simulink model "DFADAS2_SenFus_v1_201204RC_training_210115"  (R2018b)
settings: Solver=FixedStepDiscrete  StartTime=0.0  StopTime=inf  FixedStep=0.002  RelTol=1e-3  EnableMultiTasking=on
PreLoadFcn:
  | RTWConfigurationCB('preloadfcn', bdroot);
libraries: canmsglib x108, simulink x48, canfdmsglib x12
(part 2 of 28)

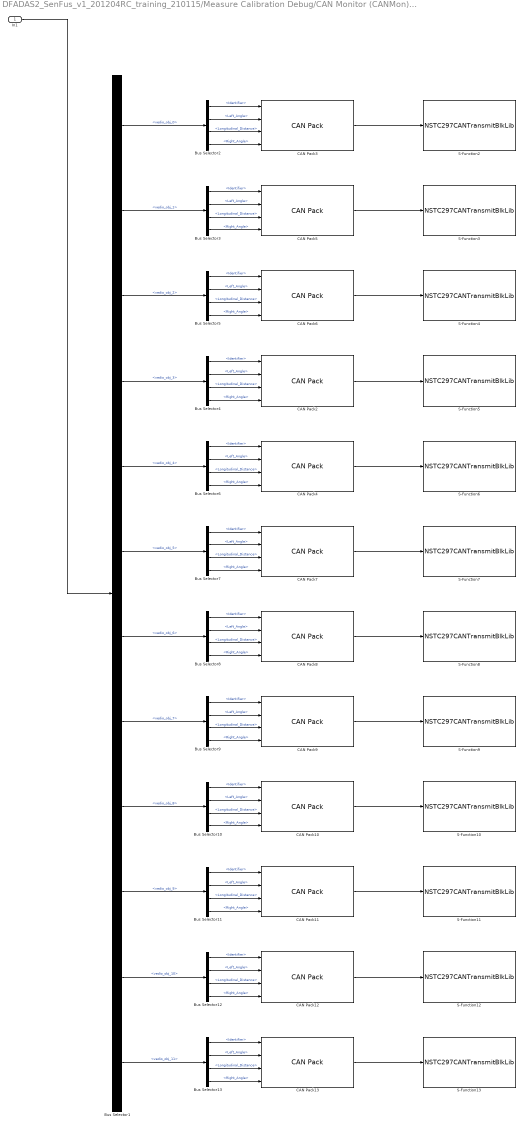
== system DFADAS2_SenFus_v1_201204RC_training_210115/Measure Calibration Debug/CAN Monitor (CANMon)/CamObjinfo ==
  In1 : Inport
  Bus Selector1 : BusSelector  OutputSignals=RawIn_bsInInfo50.EnvSens.RawObjInfo.CmrFrt.vedio_obj_0,RawIn_bsInInfo50.EnvSens.RawObjInfo.CmrFrt.vedio_obj_1,RawIn_bsInInfo50.EnvSens.RawObjInfo.CmrFrt.vedio_obj_2,RawIn_bsInInfo50.EnvSens.RawObjInfo.CmrFrt.vedio_obj_3,RawIn_bsInInfo50.EnvSens.RawObjInfo.CmrFrt.vedio_obj_4,RawIn_bsInInfo50.EnvSens.RawObjInfo.CmrFrt.vedio_obj_5,RawIn_bsInInfo50.EnvSens.RawObjInfo.CmrFrt.vedio_obj_6,RawIn_bsInInfo50.EnvSens.RawObjInfo.CmrFrt.vedio_obj_7,RawIn_bsInInfo50.EnvSens.RawObjInfo.CmrFrt.vedio_obj_8,RawIn_bsInInfo50.EnvSens.RawObjInfo.CmrFrt.vedio_obj_9,RawIn_bsInInfo50.EnvSens.RawObjInfo.CmrFrt.vedio_obj_10,RawIn_bsInInfo50.EnvSens.RawObjInfo.CmrFrt.vedio_obj_11
  Bus Selector{2..13} (12 alike) : BusSelector  OutputSignals=Identifier,Left_Angle,Longitudinal_Distance,Right_Angle
  CAN Pack10 : canmsglib/CAN Pack  CANdbFile=D:\work\ADAS ECU-Sensor CAN_V2_20190314(1).dbc  MsgList=(none)  MsgName=Video_Object_0_A  MsgIDType=Standard (11-bit identifier)  MsgIdentifier=1991  MsgLength=8  SignalInfo=Identifier_700$0$16$1$2$1$0$1$0$0$127$#Left_Angle_700$16$16$1$1$1$0$2.000000e-04$0$-8.192000e-01$8.190000e-01$#Longitudinal_Distance_700$32$16$1$2$1$0$5.000000e-02$0$0$2.047500e+02$#Right_Angle_700$48$16$1$1$1$0$2.000000e-04$0$-8.192000e-01$8.190000e-01$#  NSignals=4  StartBits=str2num('[int32(0);int32(16);int32(32);int32(48)]')  SignalSizes=str2num('[int32(16);int32(16);int32(16);int32(16)]')  ByteOrders=str2num('[int32(1);int32(1);int32(1);int32(1)]')  DataTypes=str2num('[int32(2);int32(1);int32(2);int32(1)]')  MultiplexTypes=str2num('[int32(1);int32(1);int32(1);int32(1)]')  MultiplexValues=str2num('[double(0);double(0);double(0);double(0)]')  Factors=str2num('[double(1);double(2.000000e-04);double(5.000000e-02);double(2.000000e-04)]')  Offsets=str2num('[double(0);double(0);double(0);double(0)]')  Minimums=str2num('[double(0);double(-8.192000e-01);double(0);double(-8.192000e-01)]')  Maximums=str2num('[double(127);double(8.190000e-01);double(2.047500e+02);double(8.190000e-01)]')  Remote=off  ApplyMinMax=off  BusOutput=on
      settings: SourceProductName=Simulink Real-Time  SourceProductBaseCode=XP  DataFormat=manually specified signals
  CAN Pack11 : canmsglib/CAN Pack  CANdbFile=D:\work\ADAS ECU-Sensor CAN_V2_20190314(1).dbc  MsgList=(none)  MsgName=Video_Object_0_A  MsgIDType=Standard (11-bit identifier)  MsgIdentifier=1990  MsgLength=8  SignalInfo=Identifier_700$0$16$1$2$1$0$1$0$0$127$#Left_Angle_700$16$16$1$1$1$0$2.000000e-04$0$-8.192000e-01$8.190000e-01$#Longitudinal_Distance_700$32$16$1$2$1$0$5.000000e-02$0$0$2.047500e+02$#Right_Angle_700$48$16$1$1$1$0$2.000000e-04$0$-8.192000e-01$8.190000e-01$#  NSignals=4  StartBits=str2num('[int32(0);int32(16);int32(32);int32(48)]')  SignalSizes=str2num('[int32(16);int32(16);int32(16);int32(16)]')  ByteOrders=str2num('[int32(1);int32(1);int32(1);int32(1)]')  DataTypes=str2num('[int32(2);int32(1);int32(2);int32(1)]')  MultiplexTypes=str2num('[int32(1);int32(1);int32(1);int32(1)]')  MultiplexValues=str2num('[double(0);double(0);double(0);double(0)]')  Factors=str2num('[double(1);double(2.000000e-04);double(5.000000e-02);double(2.000000e-04)]')  Offsets=str2num('[double(0);double(0);double(0);double(0)]')  Minimums=str2num('[double(0);double(-8.192000e-01);double(0);double(-8.192000e-01)]')  Maximums=str2num('[double(127);double(8.190000e-01);double(2.047500e+02);double(8.190000e-01)]')  Remote=off  ApplyMinMax=off  BusOutput=on
      settings: SourceProductName=Simulink Real-Time  SourceProductBaseCode=XP  DataFormat=manually specified signals
  CAN Pack12 : canmsglib/CAN Pack  CANdbFile=D:\work\ADAS ECU-Sensor CAN_V2_20190314(1).dbc  MsgList=(none)  MsgName=Video_Object_0_A  MsgIDType=Standard (11-bit identifier)  MsgIdentifier=1989  MsgLength=8  SignalInfo=Identifier_700$0$16$1$2$1$0$1$0$0$127$#Left_Angle_700$16$16$1$1$1$0$2.000000e-04$0$-8.192000e-01$8.190000e-01$#Longitudinal_Distance_700$32$16$1$2$1$0$5.000000e-02$0$0$2.047500e+02$#Right_Angle_700$48$16$1$1$1$0$2.000000e-04$0$-8.192000e-01$8.190000e-01$#  NSignals=4  StartBits=str2num('[int32(0);int32(16);int32(32);int32(48)]')  SignalSizes=str2num('[int32(16);int32(16);int32(16);int32(16)]')  ByteOrders=str2num('[int32(1);int32(1);int32(1);int32(1)]')  DataTypes=str2num('[int32(2);int32(1);int32(2);int32(1)]')  MultiplexTypes=str2num('[int32(1);int32(1);int32(1);int32(1)]')  MultiplexValues=str2num('[double(0);double(0);double(0);double(0)]')  Factors=str2num('[double(1);double(2.000000e-04);double(5.000000e-02);double(2.000000e-04)]')  Offsets=str2num('[double(0);double(0);double(0);double(0)]')  Minimums=str2num('[double(0);double(-8.192000e-01);double(0);double(-8.192000e-01)]')  Maximums=str2num('[double(127);double(8.190000e-01);double(2.047500e+02);double(8.190000e-01)]')  Remote=off  ApplyMinMax=off  BusOutput=on
      settings: SourceProductName=Simulink Real-Time  SourceProductBaseCode=XP  DataFormat=manually specified signals
  CAN Pack13 : canmsglib/CAN Pack  CANdbFile=D:\work\ADAS ECU-Sensor CAN_V2_20190314(1).dbc  MsgList=(none)  MsgName=Video_Object_0_A  MsgIDType=Standard (11-bit identifier)  MsgIdentifier=1988  MsgLength=8  SignalInfo=Identifier_700$0$16$1$2$1$0$1$0$0$127$#Left_Angle_700$16$16$1$1$1$0$2.000000e-04$0$-8.192000e-01$8.190000e-01$#Longitudinal_Distance_700$32$16$1$2$1$0$5.000000e-02$0$0$2.047500e+02$#Right_Angle_700$48$16$1$1$1$0$2.000000e-04$0$-8.192000e-01$8.190000e-01$#  NSignals=4  StartBits=str2num('[int32(0);int32(16);int32(32);int32(48)]')  SignalSizes=str2num('[int32(16);int32(16);int32(16);int32(16)]')  ByteOrders=str2num('[int32(1);int32(1);int32(1);int32(1)]')  DataTypes=str2num('[int32(2);int32(1);int32(2);int32(1)]')  MultiplexTypes=str2num('[int32(1);int32(1);int32(1);int32(1)]')  MultiplexValues=str2num('[double(0);double(0);double(0);double(0)]')  Factors=str2num('[double(1);double(2.000000e-04);double(5.000000e-02);double(2.000000e-04)]')  Offsets=str2num('[double(0);double(0);double(0);double(0)]')  Minimums=str2num('[double(0);double(-8.192000e-01);double(0);double(-8.192000e-01)]')  Maximums=str2num('[double(127);double(8.190000e-01);double(2.047500e+02);double(8.190000e-01)]')  Remote=off  ApplyMinMax=off  BusOutput=on
      settings: SourceProductName=Simulink Real-Time  SourceProductBaseCode=XP  DataFormat=manually specified signals
  CAN Pack2 : canmsglib/CAN Pack  CANdbFile=D:\work\ADAS ECU-Sensor CAN_V2_20190314(1).dbc  MsgList=(none)  MsgName=Video_Object_0_A  MsgIDType=Standard (11-bit identifier)  MsgIdentifier=1996  MsgLength=8  SignalInfo=Identifier_700$0$16$1$2$1$0$1$0$0$127$#Left_Angle_700$16$16$1$1$1$0$2.000000e-04$0$-8.192000e-01$8.190000e-01$#Longitudinal_Distance_700$32$16$1$2$1$0$5.000000e-02$0$0$2.047500e+02$#Right_Angle_700$48$16$1$1$1$0$2.000000e-04$0$-8.192000e-01$8.190000e-01$#  NSignals=4  StartBits=str2num('[int32(0);int32(16);int32(32);int32(48)]')  SignalSizes=str2num('[int32(16);int32(16);int32(16);int32(16)]')  ByteOrders=str2num('[int32(1);int32(1);int32(1);int32(1)]')  DataTypes=str2num('[int32(2);int32(1);int32(2);int32(1)]')  MultiplexTypes=str2num('[int32(1);int32(1);int32(1);int32(1)]')  MultiplexValues=str2num('[double(0);double(0);double(0);double(0)]')  Factors=str2num('[double(1);double(2.000000e-04);double(5.000000e-02);double(2.000000e-04)]')  Offsets=str2num('[double(0);double(0);double(0);double(0)]')  Minimums=str2num('[double(0);double(-8.192000e-01);double(0);double(-8.192000e-01)]')  Maximums=str2num('[double(127);double(8.190000e-01);double(2.047500e+02);double(8.190000e-01)]')  Remote=off  ApplyMinMax=off  BusOutput=on
      settings: SourceProductName=Simulink Real-Time  SourceProductBaseCode=XP  DataFormat=manually specified signals
  CAN Pack3 : canmsglib/CAN Pack  CANdbFile=D:\work\ADAS ECU-Sensor CAN_V2_20190314(1).dbc  MsgList=(none)  MsgName=Video_Object_0_A  MsgIDType=Standard (11-bit identifier)  MsgIdentifier=1999  MsgLength=8  SignalInfo=Identifier_700$0$16$1$2$1$0$1$0$0$127$#Left_Angle_700$16$16$1$1$1$0$2.000000e-04$0$-8.192000e-01$8.190000e-01$#Longitudinal_Distance_700$32$16$1$2$1$0$5.000000e-02$0$0$2.047500e+02$#Right_Angle_700$48$16$1$1$1$0$2.000000e-04$0$-8.192000e-01$8.190000e-01$#  NSignals=4  StartBits=str2num('[int32(0);int32(16);int32(32);int32(48)]')  SignalSizes=str2num('[int32(16);int32(16);int32(16);int32(16)]')  ByteOrders=str2num('[int32(1);int32(1);int32(1);int32(1)]')  DataTypes=str2num('[int32(2);int32(1);int32(2);int32(1)]')  MultiplexTypes=str2num('[int32(1);int32(1);int32(1);int32(1)]')  MultiplexValues=str2num('[double(0);double(0);double(0);double(0)]')  Factors=str2num('[double(1);double(2.000000e-04);double(5.000000e-02);double(2.000000e-04)]')  Offsets=str2num('[double(0);double(0);double(0);double(0)]')  Minimums=str2num('[double(0);double(-8.192000e-01);double(0);double(-8.192000e-01)]')  Maximums=str2num('[double(127);double(8.190000e-01);double(2.047500e+02);double(8.190000e-01)]')  Remote=off  ApplyMinMax=off  BusOutput=on
      settings: SourceProductName=Simulink Real-Time  SourceProductBaseCode=XP  DataFormat=manually specified signals
  CAN Pack4 : canmsglib/CAN Pack  CANdbFile=D:\work\ADAS ECU-Sensor CAN_V2_20190314(1).dbc  MsgList=(none)  MsgName=Video_Object_0_A  MsgIDType=Standard (11-bit identifier)  MsgIdentifier=1995  MsgLength=8  SignalInfo=Identifier_700$0$16$1$2$1$0$1$0$0$127$#Left_Angle_700$16$16$1$1$1$0$2.000000e-04$0$-8.192000e-01$8.190000e-01$#Longitudinal_Distance_700$32$16$1$2$1$0$5.000000e-02$0$0$2.047500e+02$#Right_Angle_700$48$16$1$1$1$0$2.000000e-04$0$-8.192000e-01$8.190000e-01$#  NSignals=4  StartBits=str2num('[int32(0);int32(16);int32(32);int32(48)]')  SignalSizes=str2num('[int32(16);int32(16);int32(16);int32(16)]')  ByteOrders=str2num('[int32(1);int32(1);int32(1);int32(1)]')  DataTypes=str2num('[int32(2);int32(1);int32(2);int32(1)]')  MultiplexTypes=str2num('[int32(1);int32(1);int32(1);int32(1)]')  MultiplexValues=str2num('[double(0);double(0);double(0);double(0)]')  Factors=str2num('[double(1);double(2.000000e-04);double(5.000000e-02);double(2.000000e-04)]')  Offsets=str2num('[double(0);double(0);double(0);double(0)]')  Minimums=str2num('[double(0);double(-8.192000e-01);double(0);double(-8.192000e-01)]')  Maximums=str2num('[double(127);double(8.190000e-01);double(2.047500e+02);double(8.190000e-01)]')  Remote=off  ApplyMinMax=off  BusOutput=on
      settings: SourceProductName=Simulink Real-Time  SourceProductBaseCode=XP  DataFormat=manually specified signals
  CAN Pack5 : canmsglib/CAN Pack  CANdbFile=D:\work\ADAS ECU-Sensor CAN_V2_20190314(1).dbc  MsgList=(none)  MsgName=Video_Object_0_A  MsgIDType=Standard (11-bit identifier)  MsgIdentifier=1998  MsgLength=8  SignalInfo=Identifier_700$0$16$1$2$1$0$1$0$0$127$#Left_Angle_700$16$16$1$1$1$0$2.000000e-04$0$-8.192000e-01$8.190000e-01$#Longitudinal_Distance_700$32$16$1$2$1$0$5.000000e-02$0$0$2.047500e+02$#Right_Angle_700$48$16$1$1$1$0$2.000000e-04$0$-8.192000e-01$8.190000e-01$#  NSignals=4  StartBits=str2num('[int32(0);int32(16);int32(32);int32(48)]')  SignalSizes=str2num('[int32(16);int32(16);int32(16);int32(16)]')  ByteOrders=str2num('[int32(1);int32(1);int32(1);int32(1)]')  DataTypes=str2num('[int32(2);int32(1);int32(2);int32(1)]')  MultiplexTypes=str2num('[int32(1);int32(1);int32(1);int32(1)]')  MultiplexValues=str2num('[double(0);double(0);double(0);double(0)]')  Factors=str2num('[double(1);double(2.000000e-04);double(5.000000e-02);double(2.000000e-04)]')  Offsets=str2num('[double(0);double(0);double(0);double(0)]')  Minimums=str2num('[double(0);double(-8.192000e-01);double(0);double(-8.192000e-01)]')  Maximums=str2num('[double(127);double(8.190000e-01);double(2.047500e+02);double(8.190000e-01)]')  Remote=off  ApplyMinMax=off  BusOutput=on
      settings: SourceProductName=Simulink Real-Time  SourceProductBaseCode=XP  DataFormat=manually specified signals
  CAN Pack6 : canmsglib/CAN Pack  CANdbFile=D:\work\ADAS ECU-Sensor CAN_V2_20190314(1).dbc  MsgList=(none)  MsgName=Video_Object_0_A  MsgIDType=Standard (11-bit identifier)  MsgIdentifier=1997  MsgLength=8  SignalInfo=Identifier_700$0$16$1$2$1$0$1$0$0$127$#Left_Angle_700$16$16$1$1$1$0$2.000000e-04$0$-8.192000e-01$8.190000e-01$#Longitudinal_Distance_700$32$16$1$2$1$0$5.000000e-02$0$0$2.047500e+02$#Right_Angle_700$48$16$1$1$1$0$2.000000e-04$0$-8.192000e-01$8.190000e-01$#  NSignals=4  StartBits=str2num('[int32(0);int32(16);int32(32);int32(48)]')  SignalSizes=str2num('[int32(16);int32(16);int32(16);int32(16)]')  ByteOrders=str2num('[int32(1);int32(1);int32(1);int32(1)]')  DataTypes=str2num('[int32(2);int32(1);int32(2);int32(1)]')  MultiplexTypes=str2num('[int32(1);int32(1);int32(1);int32(1)]')  MultiplexValues=str2num('[double(0);double(0);double(0);double(0)]')  Factors=str2num('[double(1);double(2.000000e-04);double(5.000000e-02);double(2.000000e-04)]')  Offsets=str2num('[double(0);double(0);double(0);double(0)]')  Minimums=str2num('[double(0);double(-8.192000e-01);double(0);double(-8.192000e-01)]')  Maximums=str2num('[double(127);double(8.190000e-01);double(2.047500e+02);double(8.190000e-01)]')  Remote=off  ApplyMinMax=off  BusOutput=on
      settings: SourceProductName=Simulink Real-Time  SourceProductBaseCode=XP  DataFormat=manually specified signals
  CAN Pack7 : canmsglib/CAN Pack  CANdbFile=D:\work\ADAS ECU-Sensor CAN_V2_20190314(1).dbc  MsgList=(none)  MsgName=Video_Object_0_A  MsgIDType=Standard (11-bit identifier)  MsgIdentifier=1994  MsgLength=8  SignalInfo=Identifier_700$0$16$1$2$1$0$1$0$0$127$#Left_Angle_700$16$16$1$1$1$0$2.000000e-04$0$-8.192000e-01$8.190000e-01$#Longitudinal_Distance_700$32$16$1$2$1$0$5.000000e-02$0$0$2.047500e+02$#Right_Angle_700$48$16$1$1$1$0$2.000000e-04$0$-8.192000e-01$8.190000e-01$#  NSignals=4  StartBits=str2num('[int32(0);int32(16);int32(32);int32(48)]')  SignalSizes=str2num('[int32(16);int32(16);int32(16);int32(16)]')  ByteOrders=str2num('[int32(1);int32(1);int32(1);int32(1)]')  DataTypes=str2num('[int32(2);int32(1);int32(2);int32(1)]')  MultiplexTypes=str2num('[int32(1);int32(1);int32(1);int32(1)]')  MultiplexValues=str2num('[double(0);double(0);double(0);double(0)]')  Factors=str2num('[double(1);double(2.000000e-04);double(5.000000e-02);double(2.000000e-04)]')  Offsets=str2num('[double(0);double(0);double(0);double(0)]')  Minimums=str2num('[double(0);double(-8.192000e-01);double(0);double(-8.192000e-01)]')  Maximums=str2num('[double(127);double(8.190000e-01);double(2.047500e+02);double(8.190000e-01)]')  Remote=off  ApplyMinMax=off  BusOutput=on
      settings: SourceProductName=Simulink Real-Time  SourceProductBaseCode=XP  DataFormat=manually specified signals
  CAN Pack8 : canmsglib/CAN Pack  CANdbFile=D:\work\ADAS ECU-Sensor CAN_V2_20190314(1).dbc  MsgList=(none)  MsgName=Video_Object_0_A  MsgIDType=Standard (11-bit identifier)  MsgIdentifier=1993  MsgLength=8  SignalInfo=Identifier_700$0$16$1$2$1$0$1$0$0$127$#Left_Angle_700$16$16$1$1$1$0$2.000000e-04$0$-8.192000e-01$8.190000e-01$#Longitudinal_Distance_700$32$16$1$2$1$0$5.000000e-02$0$0$2.047500e+02$#Right_Angle_700$48$16$1$1$1$0$2.000000e-04$0$-8.192000e-01$8.190000e-01$#  NSignals=4  StartBits=str2num('[int32(0);int32(16);int32(32);int32(48)]')  SignalSizes=str2num('[int32(16);int32(16);int32(16);int32(16)]')  ByteOrders=str2num('[int32(1);int32(1);int32(1);int32(1)]')  DataTypes=str2num('[int32(2);int32(1);int32(2);int32(1)]')  MultiplexTypes=str2num('[int32(1);int32(1);int32(1);int32(1)]')  MultiplexValues=str2num('[double(0);double(0);double(0);double(0)]')  Factors=str2num('[double(1);double(2.000000e-04);double(5.000000e-02);double(2.000000e-04)]')  Offsets=str2num('[double(0);double(0);double(0);double(0)]')  Minimums=str2num('[double(0);double(-8.192000e-01);double(0);double(-8.192000e-01)]')  Maximums=str2num('[double(127);double(8.190000e-01);double(2.047500e+02);double(8.190000e-01)]')  Remote=off  ApplyMinMax=off  BusOutput=on
      settings: SourceProductName=Simulink Real-Time  SourceProductBaseCode=XP  DataFormat=manually specified signals
  CAN Pack9 : canmsglib/CAN Pack  CANdbFile=D:\work\ADAS ECU-Sensor CAN_V2_20190314(1).dbc  MsgList=(none)  MsgName=Video_Object_0_A  MsgIDType=Standard (11-bit identifier)  MsgIdentifier=1992  MsgLength=8  SignalInfo=Identifier_700$0$16$1$2$1$0$1$0$0$127$#Left_Angle_700$16$16$1$1$1$0$2.000000e-04$0$-8.192000e-01$8.190000e-01$#Longitudinal_Distance_700$32$16$1$2$1$0$5.000000e-02$0$0$2.047500e+02$#Right_Angle_700$48$16$1$1$1$0$2.000000e-04$0$-8.192000e-01$8.190000e-01$#  NSignals=4  StartBits=str2num('[int32(0);int32(16);int32(32);int32(48)]')  SignalSizes=str2num('[int32(16);int32(16);int32(16);int32(16)]')  ByteOrders=str2num('[int32(1);int32(1);int32(1);int32(1)]')  DataTypes=str2num('[int32(2);int32(1);int32(2);int32(1)]')  MultiplexTypes=str2num('[int32(1);int32(1);int32(1);int32(1)]')  MultiplexValues=str2num('[double(0);double(0);double(0);double(0)]')  Factors=str2num('[double(1);double(2.000000e-04);double(5.000000e-02);double(2.000000e-04)]')  Offsets=str2num('[double(0);double(0);double(0);double(0)]')  Minimums=str2num('[double(0);double(-8.192000e-01);double(0);double(-8.192000e-01)]')  Maximums=str2num('[double(127);double(8.190000e-01);double(2.047500e+02);double(8.190000e-01)]')  Remote=off  ApplyMinMax=off  BusOutput=on
      settings: SourceProductName=Simulink Real-Time  SourceProductBaseCode=XP  DataFormat=manually specified signals
  S-Function10 : S-Function  FunctionName=NSTC297CANTransmitBlkLib  Parameters=|  SFunctionDeploymentMode=off  EnableBusSupport=off  mask(NSTC297 CAN Transmit){Ns_DeviceID=General Control Unit Gen2, Ns_ChannelNum=0, Ns_FrameType=CAN, Ns_FrameBufferSize=0, Ns_OverflowCntOutFlg=off, Ns_SampleTime=0.05}
      | uint16(Ns_DeviceID),
      | uint16(Ns_ChannelNum),
      | uint16(Ns_FrameType),
      | uint16(Ns_FrameBufferSize),
      | uint8(Ns_OverflowCntOutFlg),
      | double(Ns_SampleTime)
      mask prompts: Ns_DeviceID "Device:"; Ns_ChannelNum "Channel number:"; Ns_FrameType "Frame type:"; Ns_FrameBufferSize "Frame buffer size:"; Ns_OverflowCntOutFlg "Overflow count output"; Ns_SampleTime "Sample time:"
      mask init:
      | NSTC297CANTransmit_callback('portlabels');
      mask TypeOptions Ns_DeviceID: General Control Unit Gen2 | ADAS Control Unit Gen2
      mask TypeOptions Ns_ChannelNum: 0 | 1 | 2 | 3 | 4 | 5
      mask TypeOptions Ns_FrameType: CAN | CANFD
      mask Display: color('blue');text(0.98,0.9,'NovSteeds TC297','horizontalAlignment','right');color('blue');text(0.5,0.65,'CAN Transmit','horizontalAlignment','center');color('black');text(0.5,0.35,'Type: CAN','horizontalAlignment','center');text(0.5,0.50,'Channel: 0','horizontalAlignment','center');port_label('input',1, 'Msg');
  S-Function11 : S-Function  FunctionName=NSTC297CANTransmitBlkLib  Parameters=|  SFunctionDeploymentMode=off  EnableBusSupport=off  mask(NSTC297 CAN Transmit){Ns_DeviceID=General Control Unit Gen2, Ns_ChannelNum=0, Ns_FrameType=CAN, Ns_FrameBufferSize=0, Ns_OverflowCntOutFlg=off, Ns_SampleTime=0.05}
      | uint16(Ns_DeviceID),
      | uint16(Ns_ChannelNum),
      | uint16(Ns_FrameType),
      | uint16(Ns_FrameBufferSize),
      | uint8(Ns_OverflowCntOutFlg),
      | double(Ns_SampleTime)
      mask prompts: Ns_DeviceID "Device:"; Ns_ChannelNum "Channel number:"; Ns_FrameType "Frame type:"; Ns_FrameBufferSize "Frame buffer size:"; Ns_OverflowCntOutFlg "Overflow count output"; Ns_SampleTime "Sample time:"
      mask init:
      | NSTC297CANTransmit_callback('portlabels');
      mask TypeOptions Ns_DeviceID: General Control Unit Gen2 | ADAS Control Unit Gen2
      mask TypeOptions Ns_ChannelNum: 0 | 1 | 2 | 3 | 4 | 5
      mask TypeOptions Ns_FrameType: CAN | CANFD
      mask Display: color('blue');text(0.98,0.9,'NovSteeds TC297','horizontalAlignment','right');color('blue');text(0.5,0.65,'CAN Transmit','horizontalAlignment','center');color('black');text(0.5,0.35,'Type: CAN','horizontalAlignment','center');text(0.5,0.50,'Channel: 0','horizontalAlignment','center');port_label('input',1, 'Msg');
  S-Function12 : S-Function  FunctionName=NSTC297CANTransmitBlkLib  Parameters=|  SFunctionDeploymentMode=off  EnableBusSupport=off  mask(NSTC297 CAN Transmit){Ns_DeviceID=General Control Unit Gen2, Ns_ChannelNum=0, Ns_FrameType=CAN, Ns_FrameBufferSize=0, Ns_OverflowCntOutFlg=off, Ns_SampleTime=0.05}
      | uint16(Ns_DeviceID),
      | uint16(Ns_ChannelNum),
      | uint16(Ns_FrameType),
      | uint16(Ns_FrameBufferSize),
      | uint8(Ns_OverflowCntOutFlg),
      | double(Ns_SampleTime)
      mask prompts: Ns_DeviceID "Device:"; Ns_ChannelNum "Channel number:"; Ns_FrameType "Frame type:"; Ns_FrameBufferSize "Frame buffer size:"; Ns_OverflowCntOutFlg "Overflow count output"; Ns_SampleTime "Sample time:"
      mask init:
      | NSTC297CANTransmit_callback('portlabels');
      mask TypeOptions Ns_DeviceID: General Control Unit Gen2 | ADAS Control Unit Gen2
      mask TypeOptions Ns_ChannelNum: 0 | 1 | 2 | 3 | 4 | 5
      mask TypeOptions Ns_FrameType: CAN | CANFD
      mask Display: color('blue');text(0.98,0.9,'NovSteeds TC297','horizontalAlignment','right');color('blue');text(0.5,0.65,'CAN Transmit','horizontalAlignment','center');color('black');text(0.5,0.35,'Type: CAN','horizontalAlignment','center');text(0.5,0.50,'Channel: 0','horizontalAlignment','center');port_label('input',1, 'Msg');
  S-Function13 : S-Function  FunctionName=NSTC297CANTransmitBlkLib  Parameters=|  SFunctionDeploymentMode=off  EnableBusSupport=off  mask(NSTC297 CAN Transmit){Ns_DeviceID=General Control Unit Gen2, Ns_ChannelNum=0, Ns_FrameType=CAN, Ns_FrameBufferSize=0, Ns_OverflowCntOutFlg=off, Ns_SampleTime=0.05}
      | uint16(Ns_DeviceID),
      | uint16(Ns_ChannelNum),
      | uint16(Ns_FrameType),
      | uint16(Ns_FrameBufferSize),
      | uint8(Ns_OverflowCntOutFlg),
      | double(Ns_SampleTime)
      mask prompts: Ns_DeviceID "Device:"; Ns_ChannelNum "Channel number:"; Ns_FrameType "Frame type:"; Ns_FrameBufferSize "Frame buffer size:"; Ns_OverflowCntOutFlg "Overflow count output"; Ns_SampleTime "Sample time:"
      mask init:
      | NSTC297CANTransmit_callback('portlabels');
      mask TypeOptions Ns_DeviceID: General Control Unit Gen2 | ADAS Control Unit Gen2
      mask TypeOptions Ns_ChannelNum: 0 | 1 | 2 | 3 | 4 | 5
      mask TypeOptions Ns_FrameType: CAN | CANFD
      mask Display: color('blue');text(0.98,0.9,'NovSteeds TC297','horizontalAlignment','right');color('blue');text(0.5,0.65,'CAN Transmit','horizontalAlignment','center');color('black');text(0.5,0.35,'Type: CAN','horizontalAlignment','center');text(0.5,0.50,'Channel: 0','horizontalAlignment','center');port_label('input',1, 'Msg');
  S-Function2 : S-Function  FunctionName=NSTC297CANTransmitBlkLib  Parameters=|  SFunctionDeploymentMode=off  EnableBusSupport=off  mask(NSTC297 CAN Transmit){Ns_DeviceID=General Control Unit Gen2, Ns_ChannelNum=0, Ns_FrameType=CAN, Ns_FrameBufferSize=0, Ns_OverflowCntOutFlg=off, Ns_SampleTime=0.05}
      | uint16(Ns_DeviceID),
      | uint16(Ns_ChannelNum),
      | uint16(Ns_FrameType),
      | uint16(Ns_FrameBufferSize),
      | uint8(Ns_OverflowCntOutFlg),
      | double(Ns_SampleTime)
      mask prompts: Ns_DeviceID "Device:"; Ns_ChannelNum "Channel number:"; Ns_FrameType "Frame type:"; Ns_FrameBufferSize "Frame buffer size:"; Ns_OverflowCntOutFlg "Overflow count output"; Ns_SampleTime "Sample time:"
      mask init:
      | NSTC297CANTransmit_callback('portlabels');
      mask TypeOptions Ns_DeviceID: General Control Unit Gen2 | ADAS Control Unit Gen2
      mask TypeOptions Ns_ChannelNum: 0 | 1 | 2 | 3 | 4 | 5
      mask TypeOptions Ns_FrameType: CAN | CANFD
      mask Display: color('blue');text(0.98,0.9,'NovSteeds TC297','horizontalAlignment','right');color('blue');text(0.5,0.65,'CAN Transmit','horizontalAlignment','center');color('black');text(0.5,0.35,'Type: CAN','horizontalAlignment','center');text(0.5,0.50,'Channel: 0','horizontalAlignment','center');port_label('input',1, 'Msg');
  S-Function3 : S-Function  FunctionName=NSTC297CANTransmitBlkLib  Parameters=|  SFunctionDeploymentMode=off  EnableBusSupport=off  mask(NSTC297 CAN Transmit){Ns_DeviceID=General Control Unit Gen2, Ns_ChannelNum=0, Ns_FrameType=CAN, Ns_FrameBufferSize=0, Ns_OverflowCntOutFlg=off, Ns_SampleTime=0.05}
      | uint16(Ns_DeviceID),
      | uint16(Ns_ChannelNum),
      | uint16(Ns_FrameType),
      | uint16(Ns_FrameBufferSize),
      | uint8(Ns_OverflowCntOutFlg),
      | double(Ns_SampleTime)
      mask prompts: Ns_DeviceID "Device:"; Ns_ChannelNum "Channel number:"; Ns_FrameType "Frame type:"; Ns_FrameBufferSize "Frame buffer size:"; Ns_OverflowCntOutFlg "Overflow count output"; Ns_SampleTime "Sample time:"
      mask init:
      | NSTC297CANTransmit_callback('portlabels');
      mask TypeOptions Ns_DeviceID: General Control Unit Gen2 | ADAS Control Unit Gen2
      mask TypeOptions Ns_ChannelNum: 0 | 1 | 2 | 3 | 4 | 5
      mask TypeOptions Ns_FrameType: CAN | CANFD
      mask Display: color('blue');text(0.98,0.9,'NovSteeds TC297','horizontalAlignment','right');color('blue');text(0.5,0.65,'CAN Transmit','horizontalAlignment','center');color('black');text(0.5,0.35,'Type: CAN','horizontalAlignment','center');text(0.5,0.50,'Channel: 0','horizontalAlignment','center');port_label('input',1, 'Msg');
  S-Function4 : S-Function  FunctionName=NSTC297CANTransmitBlkLib  Parameters=|  SFunctionDeploymentMode=off  EnableBusSupport=off  mask(NSTC297 CAN Transmit){Ns_DeviceID=General Control Unit Gen2, Ns_ChannelNum=0, Ns_FrameType=CAN, Ns_FrameBufferSize=0, Ns_OverflowCntOutFlg=off, Ns_SampleTime=0.05}
      | uint16(Ns_DeviceID),
      | uint16(Ns_ChannelNum),
      | uint16(Ns_FrameType),
      | uint16(Ns_FrameBufferSize),
      | uint8(Ns_OverflowCntOutFlg),
      | double(Ns_SampleTime)
      mask prompts: Ns_DeviceID "Device:"; Ns_ChannelNum "Channel number:"; Ns_FrameType "Frame type:"; Ns_FrameBufferSize "Frame buffer size:"; Ns_OverflowCntOutFlg "Overflow count output"; Ns_SampleTime "Sample time:"
      mask init:
      | NSTC297CANTransmit_callback('portlabels');
      mask TypeOptions Ns_DeviceID: General Control Unit Gen2 | ADAS Control Unit Gen2
      mask TypeOptions Ns_ChannelNum: 0 | 1 | 2 | 3 | 4 | 5
      mask TypeOptions Ns_FrameType: CAN | CANFD
      mask Display: color('blue');text(0.98,0.9,'NovSteeds TC297','horizontalAlignment','right');color('blue');text(0.5,0.65,'CAN Transmit','horizontalAlignment','center');color('black');text(0.5,0.35,'Type: CAN','horizontalAlignment','center');text(0.5,0.50,'Channel: 0','horizontalAlignment','center');port_label('input',1, 'Msg');
  S-Function5 : S-Function  FunctionName=NSTC297CANTransmitBlkLib  Parameters=|  SFunctionDeploymentMode=off  EnableBusSupport=off  mask(NSTC297 CAN Transmit){Ns_DeviceID=General Control Unit Gen2, Ns_ChannelNum=0, Ns_FrameType=CAN, Ns_FrameBufferSize=0, Ns_OverflowCntOutFlg=off, Ns_SampleTime=0.05}
      | uint16(Ns_DeviceID),
      | uint16(Ns_ChannelNum),
      | uint16(Ns_FrameType),
      | uint16(Ns_FrameBufferSize),
      | uint8(Ns_OverflowCntOutFlg),
      | double(Ns_SampleTime)
      mask prompts: Ns_DeviceID "Device:"; Ns_ChannelNum "Channel number:"; Ns_FrameType "Frame type:"; Ns_FrameBufferSize "Frame buffer size:"; Ns_OverflowCntOutFlg "Overflow count output"; Ns_SampleTime "Sample time:"
      mask init:
      | NSTC297CANTransmit_callback('portlabels');
      mask TypeOptions Ns_DeviceID: General Control Unit Gen2 | ADAS Control Unit Gen2
      mask TypeOptions Ns_ChannelNum: 0 | 1 | 2 | 3 | 4 | 5
      mask TypeOptions Ns_FrameType: CAN | CANFD
      mask Display: color('blue');text(0.98,0.9,'NovSteeds TC297','horizontalAlignment','right');color('blue');text(0.5,0.65,'CAN Transmit','horizontalAlignment','center');color('black');text(0.5,0.35,'Type: CAN','horizontalAlignment','center');text(0.5,0.50,'Channel: 0','horizontalAlignment','center');port_label('input',1, 'Msg');
  S-Function6 : S-Function  FunctionName=NSTC297CANTransmitBlkLib  Parameters=|  SFunctionDeploymentMode=off  EnableBusSupport=off  mask(NSTC297 CAN Transmit){Ns_DeviceID=General Control Unit Gen2, Ns_ChannelNum=0, Ns_FrameType=CAN, Ns_FrameBufferSize=0, Ns_OverflowCntOutFlg=off, Ns_SampleTime=0.05}
      | uint16(Ns_DeviceID),
      | uint16(Ns_ChannelNum),
      | uint16(Ns_FrameType),
      | uint16(Ns_FrameBufferSize),
      | uint8(Ns_OverflowCntOutFlg),
      | double(Ns_SampleTime)
      mask prompts: Ns_DeviceID "Device:"; Ns_ChannelNum "Channel number:"; Ns_FrameType "Frame type:"; Ns_FrameBufferSize "Frame buffer size:"; Ns_OverflowCntOutFlg "Overflow count output"; Ns_SampleTime "Sample time:"
      mask init:
      | NSTC297CANTransmit_callback('portlabels');
      mask TypeOptions Ns_DeviceID: General Control Unit Gen2 | ADAS Control Unit Gen2
      mask TypeOptions Ns_ChannelNum: 0 | 1 | 2 | 3 | 4 | 5
      mask TypeOptions Ns_FrameType: CAN | CANFD
      mask Display: color('blue');text(0.98,0.9,'NovSteeds TC297','horizontalAlignment','right');color('blue');text(0.5,0.65,'CAN Transmit','horizontalAlignment','center');color('black');text(0.5,0.35,'Type: CAN','horizontalAlignment','center');text(0.5,0.50,'Channel: 0','horizontalAlignment','center');port_label('input',1, 'Msg');
  S-Function7 : S-Function  FunctionName=NSTC297CANTransmitBlkLib  Parameters=|  SFunctionDeploymentMode=off  EnableBusSupport=off  mask(NSTC297 CAN Transmit){Ns_DeviceID=General Control Unit Gen2, Ns_ChannelNum=0, Ns_FrameType=CAN, Ns_FrameBufferSize=0, Ns_OverflowCntOutFlg=off, Ns_SampleTime=0.05}
      | uint16(Ns_DeviceID),
      | uint16(Ns_ChannelNum),
      | uint16(Ns_FrameType),
      | uint16(Ns_FrameBufferSize),
      | uint8(Ns_OverflowCntOutFlg),
      | double(Ns_SampleTime)
      mask prompts: Ns_DeviceID "Device:"; Ns_ChannelNum "Channel number:"; Ns_FrameType "Frame type:"; Ns_FrameBufferSize "Frame buffer size:"; Ns_OverflowCntOutFlg "Overflow count output"; Ns_SampleTime "Sample time:"
      mask init:
      | NSTC297CANTransmit_callback('portlabels');
      mask TypeOptions Ns_DeviceID: General Control Unit Gen2 | ADAS Control Unit Gen2
      mask TypeOptions Ns_ChannelNum: 0 | 1 | 2 | 3 | 4 | 5
      mask TypeOptions Ns_FrameType: CAN | CANFD
      mask Display: color('blue');text(0.98,0.9,'NovSteeds TC297','horizontalAlignment','right');color('blue');text(0.5,0.65,'CAN Transmit','horizontalAlignment','center');color('black');text(0.5,0.35,'Type: CAN','horizontalAlignment','center');text(0.5,0.50,'Channel: 0','horizontalAlignment','center');port_label('input',1, 'Msg');
  S-Function8 : S-Function  FunctionName=NSTC297CANTransmitBlkLib  Parameters=|  SFunctionDeploymentMode=off  EnableBusSupport=off  mask(NSTC297 CAN Transmit){Ns_DeviceID=General Control Unit Gen2, Ns_ChannelNum=0, Ns_FrameType=CAN, Ns_FrameBufferSize=0, Ns_OverflowCntOutFlg=off, Ns_SampleTime=0.05}
      | uint16(Ns_DeviceID),
      | uint16(Ns_ChannelNum),
      | uint16(Ns_FrameType),
      | uint16(Ns_FrameBufferSize),
      | uint8(Ns_OverflowCntOutFlg),
      | double(Ns_SampleTime)
      mask prompts: Ns_DeviceID "Device:"; Ns_ChannelNum "Channel number:"; Ns_FrameType "Frame type:"; Ns_FrameBufferSize "Frame buffer size:"; Ns_OverflowCntOutFlg "Overflow count output"; Ns_SampleTime "Sample time:"
      mask init:
      | NSTC297CANTransmit_callback('portlabels');
      mask TypeOptions Ns_DeviceID: General Control Unit Gen2 | ADAS Control Unit Gen2
      mask TypeOptions Ns_ChannelNum: 0 | 1 | 2 | 3 | 4 | 5
      mask TypeOptions Ns_FrameType: CAN | CANFD
      mask Display: color('blue');text(0.98,0.9,'NovSteeds TC297','horizontalAlignment','right');color('blue');text(0.5,0.65,'CAN Transmit','horizontalAlignment','center');color('black');text(0.5,0.35,'Type: CAN','horizontalAlignment','center');text(0.5,0.50,'Channel: 0','horizontalAlignment','center');port_label('input',1, 'Msg');
  S-Function9 : S-Function  FunctionName=NSTC297CANTransmitBlkLib  Parameters=|  SFunctionDeploymentMode=off  EnableBusSupport=off  mask(NSTC297 CAN Transmit){Ns_DeviceID=General Control Unit Gen2, Ns_ChannelNum=0, Ns_FrameType=CAN, Ns_FrameBufferSize=0, Ns_OverflowCntOutFlg=off, Ns_SampleTime=0.05}
      | uint16(Ns_DeviceID),
      | uint16(Ns_ChannelNum),
      | uint16(Ns_FrameType),
      | uint16(Ns_FrameBufferSize),
      | uint8(Ns_OverflowCntOutFlg),
      | double(Ns_SampleTime)
      mask prompts: Ns_DeviceID "Device:"; Ns_ChannelNum "Channel number:"; Ns_FrameType "Frame type:"; Ns_FrameBufferSize "Frame buffer size:"; Ns_OverflowCntOutFlg "Overflow count output"; Ns_SampleTime "Sample time:"
      mask init:
      | NSTC297CANTransmit_callback('portlabels');
      mask TypeOptions Ns_DeviceID: General Control Unit Gen2 | ADAS Control Unit Gen2
      mask TypeOptions Ns_ChannelNum: 0 | 1 | 2 | 3 | 4 | 5
      mask TypeOptions Ns_FrameType: CAN | CANFD
      mask Display: color('blue');text(0.98,0.9,'NovSteeds TC297','horizontalAlignment','right');color('blue');text(0.5,0.65,'CAN Transmit','horizontalAlignment','center');color('black');text(0.5,0.35,'Type: CAN','horizontalAlignment','center');text(0.5,0.50,'Channel: 0','horizontalAlignment','center');port_label('input',1, 'Msg');
  wires:
  Bus Selector12/4 -> CAN Pack12/4  "<Right_Angle>"
  Bus Selector1/2 -> Bus Selector3/1  "<vedio_obj_1>"
  Bus Selector7/3 -> CAN Pack7/3  "<Longitudinal_Distance>"
  Bus Selector1/11 -> Bus Selector12/1  "<vedio_obj_10>"
  Bus Selector12/1 -> CAN Pack12/1  "<Identifier>"
  CAN Pack2/1 -> S-Function5/1
  Bus Selector1/1 -> Bus Selector2/1  "<vedio_obj_0>"
  Bus Selector9/3 -> CAN Pack9/3  "<Longitudinal_Distance>"
  Bus Selector3/2 -> CAN Pack5/2  "<Left_Angle>"
  Bus Selector8/2 -> CAN Pack8/2  "<Left_Angle>"
  CAN Pack4/1 -> S-Function6/1
  Bus Selector10/1 -> CAN Pack10/1  "<Identifier>"
  Bus Selector4/4 -> CAN Pack2/4  "<Right_Angle>"
  CAN Pack9/1 -> S-Function9/1
  Bus Selector13/2 -> CAN Pack13/2  "<Left_Angle>"
  Bus Selector4/3 -> CAN Pack2/3  "<Longitudinal_Distance>"
  Bus Selector5/1 -> CAN Pack6/1  "<Identifier>"
  CAN Pack11/1 -> S-Function11/1
  CAN Pack8/1 -> S-Function8/1
  Bus Selector1/10 -> Bus Selector11/1  "<vedio_obj_9>"
  Bus Selector5/3 -> CAN Pack6/3  "<Longitudinal_Distance>"
  Bus Selector2/2 -> CAN Pack3/2  "<Left_Angle>"
  Bus Selector13/3 -> CAN Pack13/3  "<Longitudinal_Distance>"
  Bus Selector7/2 -> CAN Pack7/2  "<Left_Angle>"
  Bus Selector4/2 -> CAN Pack2/2  "<Left_Angle>"
  Bus Selector13/1 -> CAN Pack13/1  "<Identifier>"
  CAN Pack6/1 -> S-Function4/1
  Bus Selector6/2 -> CAN Pack4/2  "<Left_Angle>"
  Bus Selector1/6 -> Bus Selector7/1  "<vedio_obj_5>"
  Bus Selector13/4 -> CAN Pack13/4  "<Right_Angle>"
  Bus Selector5/2 -> CAN Pack6/2  "<Left_Angle>"
  Bus Selector1/3 -> Bus Selector5/1  "<vedio_obj_2>"
  Bus Selector3/4 -> CAN Pack5/4  "<Right_Angle>"
  Bus Selector2/1 -> CAN Pack3/1  "<Identifier>"
  Bus Selector1/5 -> Bus Selector6/1  "<vedio_obj_4>"
  Bus Selector3/1 -> CAN Pack5/1  "<Identifier>"
  Bus Selector6/4 -> CAN Pack4/4  "<Right_Angle>"
  Bus Selector10/4 -> CAN Pack10/4  "<Right_Angle>"
  Bus Selector11/3 -> CAN Pack11/3  "<Longitudinal_Distance>"
  Bus Selector9/1 -> CAN Pack9/1  "<Identifier>"
  Bus Selector1/7 -> Bus Selector8/1  "<vedio_obj_6>"
  CAN Pack10/1 -> S-Function10/1
  Bus Selector6/1 -> CAN Pack4/1  "<Identifier>"
  CAN Pack7/1 -> S-Function7/1
  Bus Selector1/12 -> Bus Selector13/1  "<vedio_obj_11>"
  Bus Selector12/2 -> CAN Pack12/2  "<Left_Angle>"
  Bus Selector4/1 -> CAN Pack2/1  "<Identifier>"
  Bus Selector1/4 -> Bus Selector4/1  "<vedio_obj_3>"
  Bus Selector7/4 -> CAN Pack7/4  "<Right_Angle>"
  Bus Selector6/3 -> CAN Pack4/3  "<Longitudinal_Distance>"
  Bus Selector11/4 -> CAN Pack11/4  "<Right_Angle>"
  Bus Selector3/3 -> CAN Pack5/3  "<Longitudinal_Distance>"
  Bus Selector9/4 -> CAN Pack9/4  "<Right_Angle>"
  Bus Selector1/9 -> Bus Selector10/1  "<vedio_obj_8>"
  Bus Selector5/4 -> CAN Pack6/4  "<Right_Angle>"
  Bus Selector1/8 -> Bus Selector9/1  "<vedio_obj_7>"
  Bus Selector2/4 -> CAN Pack3/4  "<Right_Angle>"
  Bus Selector2/3 -> CAN Pack3/3  "<Longitudinal_Distance>"
  Bus Selector7/1 -> CAN Pack7/1  "<Identifier>"
  Bus Selector11/2 -> CAN Pack11/2  "<Left_Angle>"
  CAN Pack12/1 -> S-Function12/1
  Bus Selector11/1 -> CAN Pack11/1  "<Identifier>"
  CAN Pack3/1 -> S-Function2/1
  Bus Selector10/2 -> CAN Pack10/2  "<Left_Angle>"
  Bus Selector12/3 -> CAN Pack12/3  "<Longitudinal_Distance>"
  Bus Selector8/3 -> CAN Pack8/3  "<Longitudinal_Distance>"
  Bus Selector10/3 -> CAN Pack10/3  "<Longitudinal_Distance>"
  Bus Selector8/4 -> CAN Pack8/4  "<Right_Angle>"
  CAN Pack13/1 -> S-Function13/1
  Bus Selector8/1 -> CAN Pack8/1  "<Identifier>"
  Bus Selector9/2 -> CAN Pack9/2  "<Left_Angle>"
  CAN Pack5/1 -> S-Function3/1
  In1/1 -> Bus Selector1/1
